simulink model "TxSteering_RxMVDR_4x4_HDL_IQ"  (R2023a)
settings: Solver=FixedStepDiscrete  StartTime=0.0  StopTime=stoptime  RelTol=1e-3
PreLoadFcn:
  | model_init
InitFcn:
  | model_init
model workspace (MAT data in the model file):
  socvcb : containers.Map (value not decoded)
values from neighbouring files (symbols this model uses):
  diagLoading = 5e-3    (= 0.005)    [model_init.m]
  dmaFIFOLength = 2^nextpow2(testSrc1.FrameLength*testSrc1.SamplesPerSymbol*2)    [model_init.m]
  fc = ConverterSampleRate*7/16    (= 860160000)    [model_init.m]
  FPGAClkRate = DataSampleRate/VectorSamplingFactor    (= 245760000)    [model_init.m]
  movavg_bitshift = nextpow2(windowSize)    [model_init.m]
  mvdrPipelineDelay = covMatDelay+movAvgDelay+matrixSolveDelay+normResponseDelay    [model_init.m]
  NCO_bits = 14    [model_init.m]
  numArrayElements = 4    [model_init.m]
  NumChan = 4    [model_init.m]
  reciprocalDelay = nextpow2(reciprocalin_dt.WordLength) + 1 + reciprocalin_dt.WordLength + 2      - strcmp(reciprocalin_dt.Signedness,'Signed') + 7    [model_init.m]
  rx_mag_delay = input_dt.WordLength + 2 + ceil(log2(NumChan)) + 1 + rx_mag_window_size    [model_init.m]
  rx_mag_inverse_delay = nextpow2(rx_mag_dt.WordLength) + 1 + rx_mag_dt.WordLength + 2 + 7    [model_init.m]
  rx_mag_sum_growth = nextpow2(rx_mag_window_size)    [model_init.m]
  rx_mag_window_size = 256    [model_init.m]
  s2mmFrameSize = testSrc1.FrameLength*testSrc1.SamplesPerSymbol*3    [model_init.m]
  testSrc1 = struct()    [model_init.m]
  testSrc2 = struct()    [model_init.m]
  windowSize = 4096    [model_init.m]
undefined symbols (not defined in the file or in its folder): Add, j, NumBits1, NumBits2, physconst, Shift
libraries: hdlsllib x29, simulink x15, embreciprocals x2, dspsrcs4 x2, dsphdlmathfun2 x1, embsystolicmatrixops x1, dsphdlsigops2 x1, commrfcorlib x1
(part 3 of 3)

== system TxSteering_RxMVDR_4x4_HDL_IQ/DUT/Rx Beamforming/MVDR HDL/Normalize Response/Set Latch ==
  S : Inport
  Logical Operator5 : Logic  Operator=OR  IconShape=distinctive  AllPortsSameDT=off  OutDataTypeStr=boolean
  Unit Delay : UnitDelay  SampleTime=-1  HasFrameUpgradeWarning=on
  Q : Outport  VectorParamsAs1DForOutWhenUnconnected=off
  wires:
  S/1 -> Logical Operator5/1
  Logical Operator5/1 -> Unit Delay/1
  Unit Delay/1 -> Logical Operator5/2, Q/1

== system TxSteering_RxMVDR_4x4_HDL_IQ/DUT/Rx Beamforming/Output Selector/PackInput/Pack Samples ==
  u : Inport
  Pack Samples Fcn : MATLAB Function  TreatAsAtomicUnit=on
  y : Outport
  wires:
  u/1 -> Pack Samples Fcn/1(u)
  Pack Samples Fcn/1(y) -> y/1

== system TxSteering_RxMVDR_4x4_HDL_IQ/DUT/Rx Beamforming/Output Selector/PackInput1/Pack Samples ==
  u : Inport
  Pack Samples Fcn : MATLAB Function  TreatAsAtomicUnit=on
  y : Outport
  wires:
  u/1 -> Pack Samples Fcn/1(u)
  Pack Samples Fcn/1(y) -> y/1

== system TxSteering_RxMVDR_4x4_HDL_IQ/DUT/Rx Beamforming/Output Selector/PackMVDR/Pack Samples ==
  u : Inport
  Pack Samples Fcn : MATLAB Function  TreatAsAtomicUnit=on
  y : Outport
  wires:
  u/1 -> Pack Samples Fcn/1(u)
  Pack Samples Fcn/1(y) -> y/1

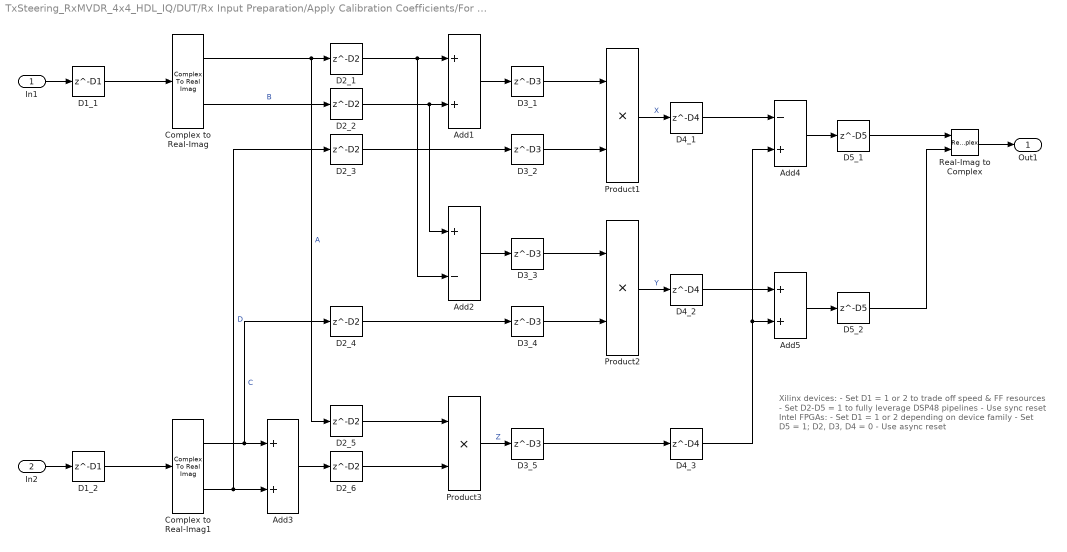
== system TxSteering_RxMVDR_4x4_HDL_IQ/DUT/Rx Input Preparation/Apply Calibration Coefficients/For Each Subsystem/HDL Complex Multiply ==
  note: Xilinx devices:
      | - Set D1 = 1 or 2 to trade off speed & FF resources
      | - Set D2-D5 = 1 to fully leverage DSP48 pipelines
      | - Use sync reset
      |
      | Intel FPGAs:
      | - Set D1 = 1 or 2 depending on device family
      | - Set D5 = 1; D2, D3, D4 = 0
      | - Use async reset
  In1 : Inport
  In2 : Inport  Port=2
  Add1 : Sum
  Add2 : Sum  Inputs=+-
  Add3 : Sum
  Add4 : Sum  Inputs=-+
  Add5 : Sum
  Complex to Real-Imag : ComplexToRealImag
  Complex to Real-Imag1 : ComplexToRealImag
  D1_1 : Delay  DelayLength=D1
  D1_2 : Delay  DelayLength=D1
  D2_{1..6} (6 alike) : Delay  DelayLength=D2
  D3_{1..5} (5 alike) : Delay  DelayLength=D3
  D4_1 : Delay  DelayLength=D4
  D4_2 : Delay  DelayLength=D4
  D4_3 : Delay  DelayLength=D4
  D5_1 : Delay  DelayLength=D5
  D5_2 : Delay  DelayLength=D5
  Product1 : Product
  Product2 : Product
  Product3 : Product
  Real-Imag to Complex : RealImagToComplex
  Out1 : Outport  VectorParamsAs1DForOutWhenUnconnected=off
  wires:
  D1_2/1 -> Complex to Real-Imag1/1
  D1_1/1 -> Complex to Real-Imag/1
  In1/1 -> D1_1/1
  D2_1/1 -> Add1/1, Add2/2
  D2_2/1 -> Add2/1, Add1/2
  D2_5/1 -> Product3/1
  D2_3/1 -> D3_2/1
  D2_4/1 -> D3_4/1
  D3_2/1 -> Product1/2
  D3_4/1 -> Product2/2
  D4_3/1 -> Add5/2, Add4/2
  D3_3/1 -> Product2/1
  D2_6/1 -> Product3/2
  D3_1/1 -> Product1/1
  Complex to Real-Imag/2 -> D2_2/1  "B"
  Complex to Real-Imag/1 -> D2_1/1, D2_5/1  "A"
  Add2/1 -> D3_3/1
  Add3/1 -> D2_6/1
  Add1/1 -> D3_1/1
  D3_5/1 -> D4_3/1
  D4_2/1 -> Add5/1
  D4_1/1 -> Add4/1
  D5_2/1 -> Real-Imag to Complex/2
  D5_1/1 -> Real-Imag to Complex/1
  Add5/1 -> D5_2/1
  Add4/1 -> D5_1/1
  Product3/1 -> D3_5/1  "Z"
  Product2/1 -> D4_2/1  "Y"
  Product1/1 -> D4_1/1  "X"
  Complex to Real-Imag1/2 -> D2_3/1, Add3/2  "D"
  Complex to Real-Imag1/1 -> D2_4/1, Add3/1  "C"
  In2/1 -> D1_2/1
  Real-Imag to Complex/1 -> Out1/1

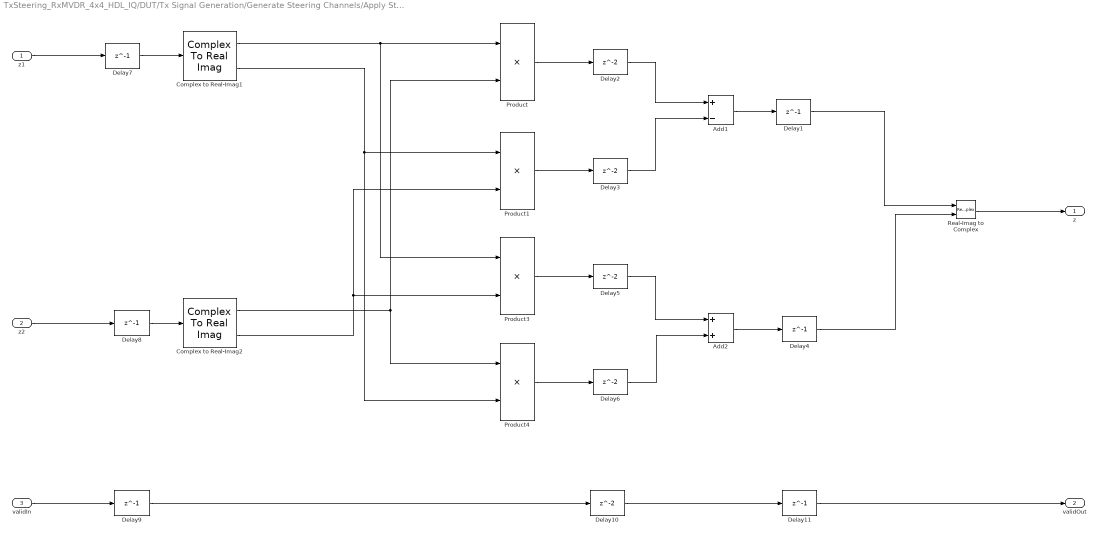
== system TxSteering_RxMVDR_4x4_HDL_IQ/DUT/Tx Signal Generation/Generate Steering Channels/Apply Steering Coefficients/HDL Complex Multiplier ==
  z1 : Inport
  z2 : Inport  Port=2
  validIn : Inport  Port=3
  Add1 : Sum  Inputs=+-
  Add2 : Sum
  Complex to Real-Imag1 : ComplexToRealImag
  Complex to Real-Imag2 : ComplexToRealImag
  Delay{1,4,7..9,11} (6 alike) : Delay  DelayLength=1  InitialCondition=0  InputProcessing=Columns as channels (frame based)
  Delay{2..3,5..6,10} (5 alike) : Delay  InitialCondition=0  InputProcessing=Columns as channels (frame based)
  Product{,1,3..4} (4 alike) : Product
  Real-Imag to Complex : RealImagToComplex
  z : Outport  VectorParamsAs1DForOutWhenUnconnected=off
  validOut : Outport  Port=2  VectorParamsAs1DForOutWhenUnconnected=off
  wires:
  Add2/1 -> Delay4/1
  Add1/1 -> Delay1/1
  Complex to Real-Imag2/2 -> Product1/2, Product3/2
  Complex to Real-Imag1/2 -> Product1/1, Product4/2
  Complex to Real-Imag2/1 -> Product/2, Product4/1
  Complex to Real-Imag1/1 -> Product/1, Product3/1
  Product/1 -> Delay2/1
  Product1/1 -> Delay3/1
  Product3/1 -> Delay5/1
  Product4/1 -> Delay6/1
  Delay2/1 -> Add1/1
  Delay3/1 -> Add1/2
  Delay6/1 -> Add2/2
  Real-Imag to Complex/1 -> z/1
  z1/1 -> Delay7/1
  z2/1 -> Delay8/1
  Delay5/1 -> Add2/1
  Delay1/1 -> Real-Imag to Complex/1
  Delay4/1 -> Real-Imag to Complex/2
  Delay7/1 -> Complex to Real-Imag1/1
  Delay8/1 -> Complex to Real-Imag2/1
  validIn/1 -> Delay9/1
  Delay9/1 -> Delay10/1
  Delay10/1 -> Delay11/1
  Delay11/1 -> validOut/1

== system TxSteering_RxMVDR_4x4_HDL_IQ/DUT/Rx Beamforming/Input Scaling/Compute Input Magnitude/Delay Enabled Synchronous/Synchronous Delay ==
  u : Inport
  E : Inport  Port=2
  Delay : Delay  DelayLength=DelayLength  InitialCondition=InitialCondition  ShowEnablePort=on
      settings: InputPortMap=u0,e6
  State Control : StateControl  StateControl=Synchronous
  y : Outport
  wires:
  Delay/1 -> y/1
  E/1 -> Delay/2
  u/1 -> Delay/1

== system TxSteering_RxMVDR_4x4_HDL_IQ/DUT/Rx Beamforming/MVDR HDL/Compute Weight Vector/Serialize Input Data/Output Selector ==
  idx : Inport
  first : Inport  Port=2
  dataIn : Inport  Port=3
  Multiport Switch : MultiPortSwitch  DataPortOrder=Zero-based contiguous  Inputs=4  zeroidx=on  SaturateOnIntegerOverflow=off  InputSameDT=off
  Row 1 : Selector  NumberOfDimensions=2  InputPortWidth=3  IndexOptions=Index vector (dialog),Select all  Indices=1,1  OutputSizes=1,1
  Row 2 : Selector  NumberOfDimensions=2  InputPortWidth=3  IndexOptions=Index vector (dialog),Select all  Indices=2,1  OutputSizes=1,1
  Row 3 : Selector  NumberOfDimensions=2  InputPortWidth=3  IndexOptions=Index vector (dialog),Select all  Indices=3,1  OutputSizes=1,1
  Row 4 : Selector  NumberOfDimensions=2  InputPortWidth=3  IndexOptions=Index vector (dialog),Select all  Indices=4,1  OutputSizes=1,1
  Unit Delay Enabled Synchronous : hdlsllib/Discrete/Unit Delay Enabled Synchronous  InitialCondition=0.0  SampleTime=-1
  dataOut : Outport
  wires:
  Row 1/1 -> Multiport Switch/2
  Row 4/1 -> Multiport Switch/5
  Unit Delay Enabled Synchronous/1 -> Row 4/1, Row 3/1, Row 2/1
  dataIn/1 -> Unit Delay Enabled Synchronous/1, Row 1/1
  Row 2/1 -> Multiport Switch/3
  idx/1 -> Multiport Switch/1
  Row 3/1 -> Multiport Switch/4
  Multiport Switch/1 -> dataOut/1
  first/1 -> Unit Delay Enabled Synchronous/2

== system TxSteering_RxMVDR_4x4_HDL_IQ/DUT/Rx Beamforming/MVDR HDL/Compute Weight Vector/Serialize Input Data/Output Selector1 ==
  idx : Inport
  first : Inport  Port=2
  dataIn : Inport  Port=3
  Multiport Switch : MultiPortSwitch  DataPortOrder=Zero-based contiguous  Inputs=4  zeroidx=on  SaturateOnIntegerOverflow=off  InputSameDT=off
  Row 1 : Selector  NumberOfDimensions=2  InputPortWidth=3  IndexOptions=Index vector (dialog),Select all  Indices=1,1  OutputSizes=1,1
  Row 2 : Selector  NumberOfDimensions=2  InputPortWidth=3  IndexOptions=Index vector (dialog),Select all  Indices=2,1  OutputSizes=1,1
  Row 3 : Selector  NumberOfDimensions=2  InputPortWidth=3  IndexOptions=Index vector (dialog),Select all  Indices=3,1  OutputSizes=1,1
  Row 4 : Selector  NumberOfDimensions=2  InputPortWidth=3  IndexOptions=Index vector (dialog),Select all  Indices=4,1  OutputSizes=1,1
  Unit Delay Enabled Synchronous : hdlsllib/Discrete/Unit Delay Enabled Synchronous  InitialCondition=0.0  SampleTime=-1
  dataOut : Outport
  wires:
  first/1 -> Unit Delay Enabled Synchronous/2
  Multiport Switch/1 -> dataOut/1
  Row 3/1 -> Multiport Switch/4
  idx/1 -> Multiport Switch/1
  Row 2/1 -> Multiport Switch/3
  dataIn/1 -> Row 1/1, Unit Delay Enabled Synchronous/1
  Unit Delay Enabled Synchronous/1 -> Row 2/1, Row 3/1, Row 4/1
  Row 4/1 -> Multiport Switch/5
  Row 1/1 -> Multiport Switch/2

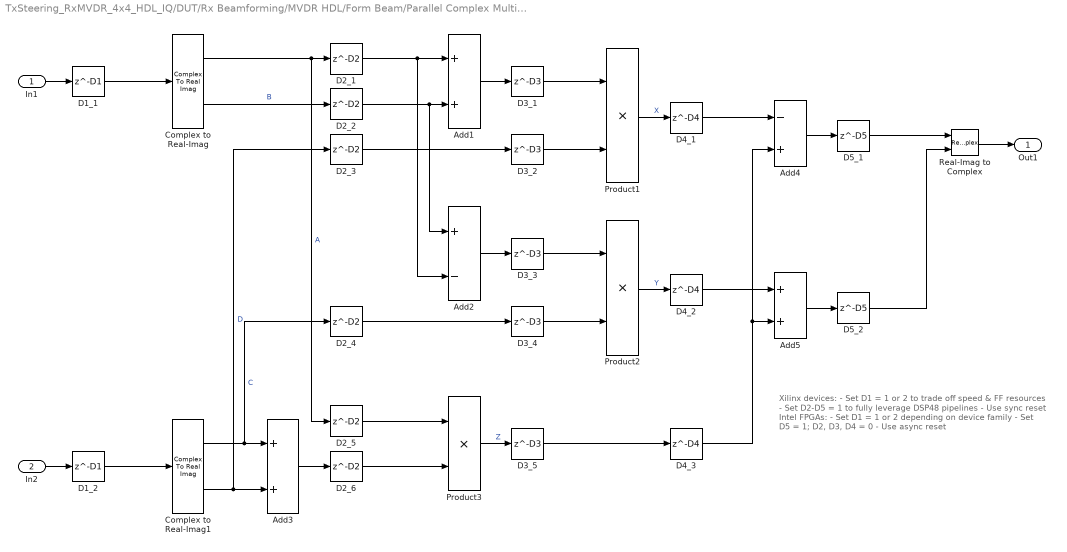
== system TxSteering_RxMVDR_4x4_HDL_IQ/DUT/Rx Beamforming/MVDR HDL/Form Beam/Parallel Complex Multiply/HDL Complex Multiply ==
  note: Xilinx devices:
      | - Set D1 = 1 or 2 to trade off speed & FF resources
      | - Set D2-D5 = 1 to fully leverage DSP48 pipelines
      | - Use sync reset
      |
      | Intel FPGAs:
      | - Set D1 = 1 or 2 depending on device family
      | - Set D5 = 1; D2, D3, D4 = 0
      | - Use async reset
  In1 : Inport
  In2 : Inport  Port=2
  Add1 : Sum
  Add2 : Sum  Inputs=+-
  Add3 : Sum
  Add4 : Sum  Inputs=-+
  Add5 : Sum
  Complex to Real-Imag : ComplexToRealImag
  Complex to Real-Imag1 : ComplexToRealImag
  D1_1 : Delay  DelayLength=D1
  D1_2 : Delay  DelayLength=D1
  D2_{1..6} (6 alike) : Delay  DelayLength=D2
  D3_{1..5} (5 alike) : Delay  DelayLength=D3
  D4_1 : Delay  DelayLength=D4
  D4_2 : Delay  DelayLength=D4
  D4_3 : Delay  DelayLength=D4
  D5_1 : Delay  DelayLength=D5
  D5_2 : Delay  DelayLength=D5
  Product1 : Product
  Product2 : Product
  Product3 : Product
  Real-Imag to Complex : RealImagToComplex
  Out1 : Outport  VectorParamsAs1DForOutWhenUnconnected=off
  wires:
  Real-Imag to Complex/1 -> Out1/1
  In2/1 -> D1_2/1
  Complex to Real-Imag1/1 -> Add3/1, D2_4/1  "C"
  Complex to Real-Imag1/2 -> Add3/2, D2_3/1  "D"
  Product1/1 -> D4_1/1  "X"
  Product2/1 -> D4_2/1  "Y"
  Product3/1 -> D3_5/1  "Z"
  Add4/1 -> D5_1/1
  Add5/1 -> D5_2/1
  D5_1/1 -> Real-Imag to Complex/1
  D5_2/1 -> Real-Imag to Complex/2
  D4_1/1 -> Add4/1
  D4_2/1 -> Add5/1
  D3_5/1 -> D4_3/1
  Add1/1 -> D3_1/1
  Add3/1 -> D2_6/1
  Add2/1 -> D3_3/1
  Complex to Real-Imag/1 -> D2_5/1, D2_1/1  "A"
  Complex to Real-Imag/2 -> D2_2/1  "B"
  D3_1/1 -> Product1/1
  D2_6/1 -> Product3/2
  D3_3/1 -> Product2/1
  D4_3/1 -> Add4/2, Add5/2
  D3_4/1 -> Product2/2
  D3_2/1 -> Product1/2
  D2_4/1 -> D3_4/1
  D2_3/1 -> D3_2/1
  D2_5/1 -> Product3/1
  D2_2/1 -> Add1/2, Add2/1
  D2_1/1 -> Add2/2, Add1/1
  In1/1 -> D1_1/1
  D1_1/1 -> Complex to Real-Imag/1
  D1_2/1 -> Complex to Real-Imag1/1

== system TxSteering_RxMVDR_4x4_HDL_IQ/DUT/Rx Beamforming/MVDR HDL/Form Covariance Matrix/Matrix Multiply Partitioned/Partition x_conj ==
  x : Inport
  x_conj : Inport  Port=2  Partition=on  PartitionDimension=1  PartitionWidth=1  PartitionOffset=0
  For Each : ForEach  DisableCoverage=on
  Partition x : Subsystem  TreatAsAtomicUnit=on
  C : Outport  ConcatenationDimension=1
  wires:
  x_conj/1 -> Partition x/2(x_conj_elem)
  x/1 -> Partition x/1(x)
  Partition x/1(C_col) -> C/1

== system TxSteering_RxMVDR_4x4_HDL_IQ/DUT/Rx Beamforming/MVDR HDL/Moving Average/Window Delay/Delay Enabled Synchronous RAM Based ==
  u : Inport
  E : Inport  Port=2
  Add : Sum  Inputs=++-  OutDataTypeStr=Inherit: Same as accumulator
  Constant1 : Constant  OutDataTypeStr=Inherit: Inherit via back propagation  SampleTime=-1
  Constant2 : Constant  Value=delay  OutDataTypeStr=Inherit: Inherit via back propagation  SampleTime=-1
  HDL Counter : hdlsllib/Sources/HDL Counter  CountType=Free running  CountInit=0  CountStep=1  CountMax=25  CountFromType=Initial value  CountFrom=0  CountResetPort=off  CountLoadPort=off  CountEnbPort=on  CountDirPort=off  CountHitOutputPort=off  CountDataType=Unsigned  CountWordLen=addrWidth  CountFracLen=0  CountSampTime=-1
  Simple Dual Port RAM System : hdlsllib/HDL RAMs/Simple Dual Port RAM System  RAMType=Simple dual port  WriteOutputValue=New data  RAMInitialValue=0  SimulateUsing=Code generation
  Switch1 : Switch  Criteria=u2 ~= 0  SaturateOnIntegerOverflow=off  InputSameDT=off
  Zero on Initial Delay : Subsystem
  out_prev : hdlsllib/Discrete/Unit Delay Enabled Synchronous  InitialCondition=0.0  SampleTime=-1
  read_prev : Delay  DelayLength=1
  y : Outport
  wires:
  read_prev/1 -> Switch1/2, out_prev/2
  Zero on Initial Delay/1(dout) -> Switch1/1, out_prev/1
  Simple Dual Port RAM System/1 -> Zero on Initial Delay/1(ram_dout)
  E/1 -> HDL Counter/1, Zero on Initial Delay/2(en), read_prev/1, Simple Dual Port RAM System/3
  out_prev/1 -> Switch1/3
  Switch1/1 -> y/1
  Constant2/1 -> Add/3
  Constant1/1 -> Add/2
  u/1 -> Simple Dual Port RAM System/1
  Add/1 -> Simple Dual Port RAM System/4
  HDL Counter/1 -> Add/1, Simple Dual Port RAM System/2

== system TxSteering_RxMVDR_4x4_HDL_IQ/DUT/Rx Beamforming/MVDR HDL/Normalize Response/MVDR Weight Update/Inner Product ==
  sv : Inport
  wp : Inport  Port=2
  validIn : Inport  Port=3
  Complex to Real-Imag : ComplexToRealImag  Output=Real
  Conjugate : Math  Operator=conj  SignedPower=on  RndMeth=Zero
  Data Type Conversion : DataTypeConversion  OutDataTypeStr=reciprocalin_dt  SaturateOnIntegerOverflow=off  RndMeth=Floor
  Delay : Delay  DelayLength=1
  Delay1 : Delay  DelayLength=6
  Delay2 : Delay  DelayLength=ceil(log2(numArrayElements))
  Delay4 : Delay  DelayLength=1
  Element-wise complex product : Subsystem  TreatAsAtomicUnit=on
  To Workspace : ToWorkspace  VariableName=norm_mag  SampleTime=-1
      settings: Save2DSignal=2-D array (concatenate along first dimension)
  To Workspace1 : ToWorkspace  VariableName=norm_mag_valid  SampleTime=-1
      settings: Save2DSignal=2-D array (concatenate along first dimension)
  Tree Sum with Distributed Pipelining : Subsystem
  y : Outport
  validOut : Outport  Port=2
  wires:
  sv/1 -> Conjugate/1
  validIn/1 -> Delay1/1
  Delay1/1 -> Delay4/1
  Delay4/1 -> Delay2/1
  wp/1 -> Element-wise complex product/1(u)
  Delay/1 -> Tree Sum with Distributed Pipelining/1(In1)
  Complex to Real-Imag/1 -> Data Type Conversion/1
  Element-wise complex product/1(y) -> Delay/1
  Delay2/1 -> validOut/1, To Workspace1/1
  Tree Sum with Distributed Pipelining/1(Out1) -> Complex to Real-Imag/1
  Data Type Conversion/1 -> y/1, To Workspace/1
  Conjugate/1 -> Element-wise complex product/2(v)

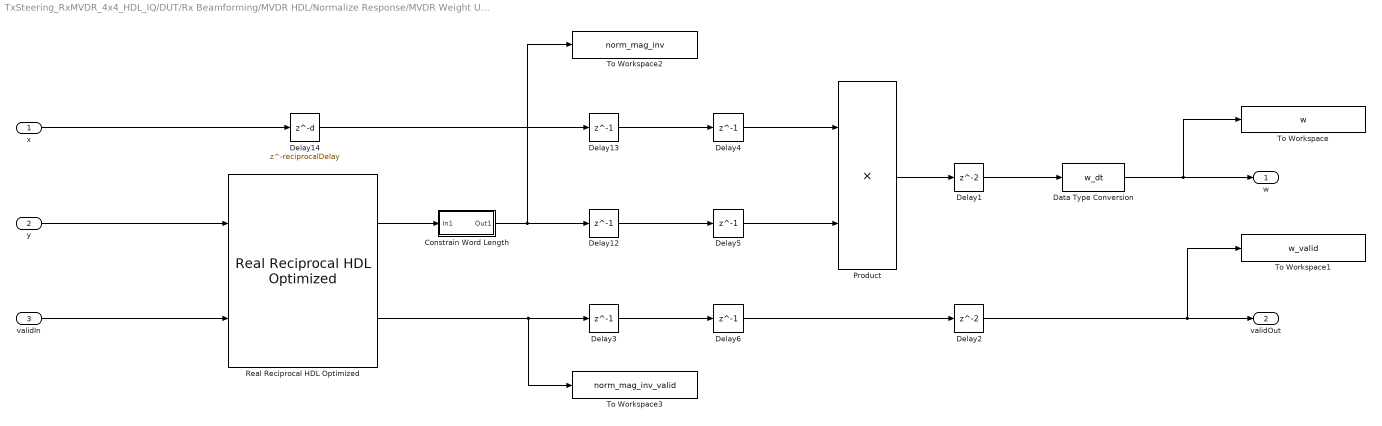
== system TxSteering_RxMVDR_4x4_HDL_IQ/DUT/Rx Beamforming/MVDR HDL/Normalize Response/MVDR Weight Update/Vector // Scalar Divide ==
  x : Inport
  y : Inport  Port=2
  validIn : Inport  Port=3
  Constrain Word Length : Subsystem  mask(Constrain Word Length){WL=18}
      mask prompts: WL "Maximum word length:"
      mask help: Output word length will not exceed the specified value.
      mask Display: fprintf('WL <= %d',WL);
  Data Type Conversion : DataTypeConversion  OutDataTypeStr=w_dt  SaturateOnIntegerOverflow=off  RndMeth=Floor
  Delay1 : Delay
  Delay{3..6,12..13} (6 alike) : Delay  DelayLength=1
  Delay14 : Delay  DelayLength=reciprocalDelay
  Delay2 : Delay
  Product : Product
  Real Reciprocal HDL Optimized : embreciprocals/Real Reciprocal HDL Optimized  OutputType=reciprocalout_dt
      settings: LibrarySourceBlock=embeddedMatrixLib/Math Operations/Real Reciprocal HDL Optimized
  To Workspace : ToWorkspace  VariableName=w  SampleTime=-1
      settings: Save2DSignal=2-D array (concatenate along first dimension)
  To Workspace1 : ToWorkspace  VariableName=w_valid  SampleTime=-1
      settings: Save2DSignal=2-D array (concatenate along first dimension)
  To Workspace2 : ToWorkspace  VariableName=norm_mag_inv  SampleTime=-1
      settings: Save2DSignal=2-D array (concatenate along first dimension)
  To Workspace3 : ToWorkspace  VariableName=norm_mag_inv_valid  SampleTime=-1
      settings: Save2DSignal=2-D array (concatenate along first dimension)
  w : Outport
  validOut : Outport  Port=2
  wires:
  y/1 -> Real Reciprocal HDL Optimized/1
  Real Reciprocal HDL Optimized/1 -> Constrain Word Length/1(In1)
  validIn/1 -> Real Reciprocal HDL Optimized/2
  Product/1 -> Delay1/1
  x/1 -> Delay14/1
  Delay14/1 -> Delay13/1
  Constrain Word Length/1(Out1) -> To Workspace2/1, Delay12/1
  Real Reciprocal HDL Optimized/2 -> To Workspace3/1, Delay3/1
  Delay2/1 -> To Workspace1/1, validOut/1
  Delay1/1 -> Data Type Conversion/1
  Data Type Conversion/1 -> To Workspace/1, w/1
  Delay4/1 -> Product/1
  Delay13/1 -> Delay4/1
  Delay5/1 -> Product/2
  Delay12/1 -> Delay5/1
  Delay3/1 -> Delay6/1
  Delay6/1 -> Delay2/1

== system TxSteering_RxMVDR_4x4_HDL_IQ/DUT/Rx Beamforming/MVDR HDL/Form Covariance Matrix/Matrix Multiply Partitioned/Partition x_conj/Partition x ==
  x : Inport  Partition=on  PartitionDimension=1  PartitionWidth=1  PartitionOffset=0
  x_conj_elem : Inport  Port=2
  For Each : ForEach  DisableCoverage=on
  HDL Complex Multiply : Subsystem  mask(HDL Complex Multiplier (3 Multiply, 5 Add)){D1=2, D2=1, D3=1, D4=1, D5=1}
      mask help:
      | Xilinx devices:
      | - Set D1 = 1 or 2 to trade off speed & FF resources
      | - Set D2-D5 = 1 to fully leverage DSP48 pipelines
      | - Use sync reset
      |
      | Intel FPGAs:
      | - Set D1 = 1 or 2 depending on device family
      | - Set D5 = 1; D2, D3, D4 = 0
      | - Use async reset
      mask init:
      | delay = D1+D2+D3+D4+D5;
      mask Display:
      | fprintf('Delay=%d',delay);
      | port_label('input',1,'z1');
      | port_label('input',2,'z2');
  C_col : Outport  ConcatenationDimension=1
  wires:
  x/1 -> HDL Complex Multiply/1(In1)
  x_conj_elem/1 -> HDL Complex Multiply/2(In2)
  HDL Complex Multiply/1(Out1) -> C_col/1

== system TxSteering_RxMVDR_4x4_HDL_IQ/DUT/Rx Beamforming/MVDR HDL/Moving Average/Window Delay/Delay Enabled Synchronous RAM Based/Zero on Initial Delay ==
  ram_dout : Inport
  en : Inport  Port=2
  AND : Logic  IconShape=distinctive  AllPortsSameDT=off  OutDataTypeStr=boolean
  Compare To Constant : simulink/Logic and Bit Operations/Compare To Constant  relop===  const=delay  OutDataTypeStr=boolean
  HDL Counter1 : hdlsllib/Sources/HDL Counter  CountType=Free running  CountInit=0  CountStep=1  CountMax=25  CountFromType=Initial value  CountFrom=0  CountResetPort=off  CountLoadPort=off  CountEnbPort=on  CountDirPort=off  CountHitOutputPort=off  CountDataType=Unsigned  CountWordLen=addrWidth  CountFracLen=0  CountSampTime=-1
  NOT : Logic  Operator=NOT  IconShape=distinctive  AllPortsSameDT=off  OutDataTypeStr=boolean
  Switch : Switch  Criteria=u2 ~= 0  SaturateOnIntegerOverflow=off  InputSameDT=off
  Zeros Like : MATLAB Function  TreatAsAtomicUnit=on  mask(Zeros Like){matchInputSize=on, outputSizeUser=[1 1]}
      mask prompts: matchInputSize "Match input size?"; outputSizeUser "Output size:"
      mask help: Creates a constant 0 signal with the same datatype as the input. Optionally match the size of the input or specify the output size.
      mask init:
      | if isscalar(outputSizeUser)
      |     outputSize = [outputSizeUser 1];
      | else
      |     outputSize = outputSizeUser;
      | end
  dout : Outport
  wires:
  en/1 -> AND/1
  ram_dout/1 -> Switch/1, Zeros Like/1(u)
  AND/1 -> HDL Counter1/1
  Zeros Like/1(y) -> Switch/3
  NOT/1 -> AND/2
  Compare To Constant/1 -> NOT/1, Switch/2
  HDL Counter1/1 -> Compare To Constant/1
  Switch/1 -> dout/1

== system TxSteering_RxMVDR_4x4_HDL_IQ/DUT/Rx Beamforming/MVDR HDL/Normalize Response/MVDR Weight Update/Inner Product/Element-wise complex product ==
  u : Inport  Partition=on  PartitionDimension=1  PartitionWidth=1  PartitionOffset=0
  v : Inport  Port=2  Partition=on  PartitionDimension=1  PartitionWidth=1  PartitionOffset=0
  For Each : ForEach  DisableCoverage=on
  HDL Complex Multiply : Subsystem  mask(HDL Complex Multiplier (3 Multiply, 5 Add)){D1=2, D2=1, D3=1, D4=1, D5=1}
      mask help:
      | Xilinx devices:
      | - Set D1 = 1 or 2 to trade off speed & FF resources
      | - Set D2-D5 = 1 to fully leverage DSP48 pipelines
      | - Use sync reset
      |
      | Intel FPGAs:
      | - Set D1 = 1 or 2 depending on device family
      | - Set D5 = 1; D2, D3, D4 = 0
      | - Use async reset
      mask init:
      | delay = D1+D2+D3+D4+D5;
      mask Display:
      | fprintf('Pipelined\nComplex Multiply\nLatency=%d',delay);
      | port_label('input',1,'z1');
      | port_label('input',2,'z2');
  y : Outport  ConcatenationDimension=1
  wires:
  v/1 -> HDL Complex Multiply/2(In2)
  u/1 -> HDL Complex Multiply/1(In1)
  HDL Complex Multiply/1(Out1) -> y/1

== system TxSteering_RxMVDR_4x4_HDL_IQ/DUT/Rx Beamforming/MVDR HDL/Normalize Response/MVDR Weight Update/Inner Product/Tree Sum with Distributed Pipelining ==
  In1 : Inport
  Delay3 : Delay  DelayLength=ceil(log2(numArrayElements))
  Tree Sum of Elements : Sum  Inputs=+  OutDataTypeStr=Inherit: Same as first input  LockScale=on
  Out1 : Outport
  wires:
  Delay3/1 -> Out1/1
  In1/1 -> Tree Sum of Elements/1
  Tree Sum of Elements/1 -> Delay3/1

== system TxSteering_RxMVDR_4x4_HDL_IQ/DUT/Rx Beamforming/MVDR HDL/Normalize Response/MVDR Weight Update/Vector // Scalar Divide/Constrain Word Length ==
  In1 : Inport
  Constant : Constant  Value=0  OutDataTypeStr=fixdt(0,WL,0)  SampleTime=-1
  Data Type Propagation : simulink/Signal Attributes/Data Type Propagation  PropDataType=fixdt(1, 16)  IfRefDouble=double  IfRefSingle=single  IsSigned=IsSigned1  NumBitsBase=min([NumBits1 NumBits2])  NumBitsMult=1  NumBitsAdd=0  NumBitsAllowFinal=1:128  PropScaling=2^-10  ValuesUsedBestPrec=[5 -7]  SlopeBase=PosRange1  SlopeMult=1  SlopeAdd=0  BiasBase=Bias1  BiasMult=1  BiasAdd=0
  Data Type Conversion : DataTypeConversion  SaturateOnIntegerOverflow=off  RndMeth=Floor
  Out1 : Outport
  wires:
  Constant/1 -> Data Type Propagation/2
  Data Type Conversion/1 -> Out1/1, Data Type Propagation/3
  In1/1 -> Data Type Conversion/1, Data Type Propagation/1

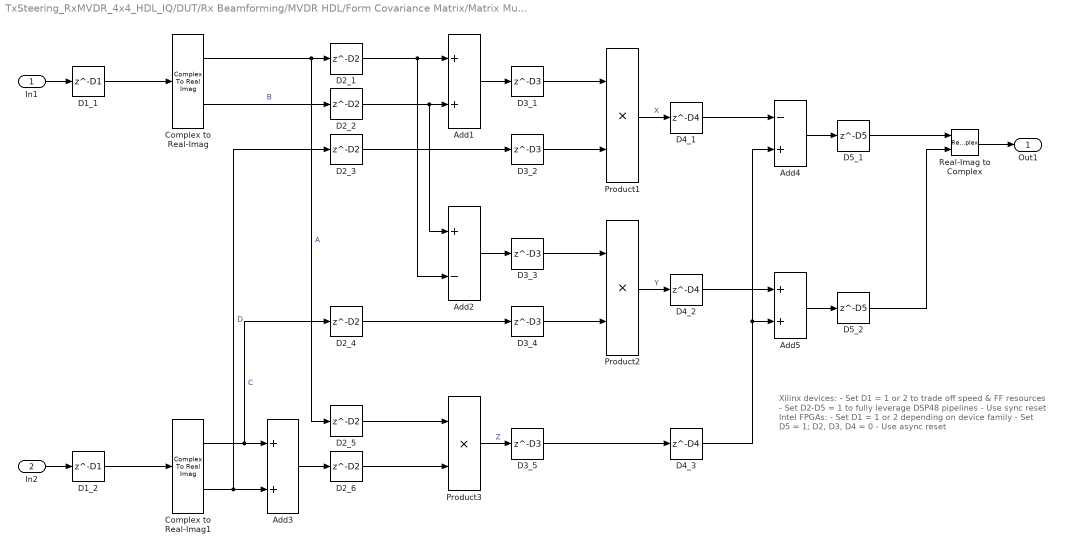
== system TxSteering_RxMVDR_4x4_HDL_IQ/DUT/Rx Beamforming/MVDR HDL/Form Covariance Matrix/Matrix Multiply Partitioned/Partition x_conj/Partition x/HDL Complex Multiply ==
  note: Xilinx devices:
      | - Set D1 = 1 or 2 to trade off speed & FF resources
      | - Set D2-D5 = 1 to fully leverage DSP48 pipelines
      | - Use sync reset
      |
      | Intel FPGAs:
      | - Set D1 = 1 or 2 depending on device family
      | - Set D5 = 1; D2, D3, D4 = 0
      | - Use async reset
  In1 : Inport
  In2 : Inport  Port=2
  Add1 : Sum
  Add2 : Sum  Inputs=+-
  Add3 : Sum
  Add4 : Sum  Inputs=-+
  Add5 : Sum
  Complex to Real-Imag : ComplexToRealImag
  Complex to Real-Imag1 : ComplexToRealImag
  D1_1 : Delay  DelayLength=D1
  D1_2 : Delay  DelayLength=D1
  D2_{1..6} (6 alike) : Delay  DelayLength=D2
  D3_{1..5} (5 alike) : Delay  DelayLength=D3
  D4_1 : Delay  DelayLength=D4
  D4_2 : Delay  DelayLength=D4
  D4_3 : Delay  DelayLength=D4
  D5_1 : Delay  DelayLength=D5
  D5_2 : Delay  DelayLength=D5
  Product1 : Product
  Product2 : Product
  Product3 : Product
  Real-Imag to Complex : RealImagToComplex
  Out1 : Outport  VectorParamsAs1DForOutWhenUnconnected=off
  wires:
  Real-Imag to Complex/1 -> Out1/1
  In2/1 -> D1_2/1
  Complex to Real-Imag1/1 -> Add3/1, D2_4/1  "C"
  Complex to Real-Imag1/2 -> Add3/2, D2_3/1  "D"
  Product1/1 -> D4_1/1  "X"
  Product2/1 -> D4_2/1  "Y"
  Product3/1 -> D3_5/1  "Z"
  Add4/1 -> D5_1/1
  Add5/1 -> D5_2/1
  D5_1/1 -> Real-Imag to Complex/1
  D5_2/1 -> Real-Imag to Complex/2
  D4_1/1 -> Add4/1
  D4_2/1 -> Add5/1
  D3_5/1 -> D4_3/1
  Add1/1 -> D3_1/1
  Add3/1 -> D2_6/1
  Add2/1 -> D3_3/1
  Complex to Real-Imag/1 -> D2_5/1, D2_1/1  "A"
  Complex to Real-Imag/2 -> D2_2/1  "B"
  D3_1/1 -> Product1/1
  D2_6/1 -> Product3/2
  D3_3/1 -> Product2/1
  D4_3/1 -> Add4/2, Add5/2
  D3_4/1 -> Product2/2
  D3_2/1 -> Product1/2
  D2_4/1 -> D3_4/1
  D2_3/1 -> D3_2/1
  D2_5/1 -> Product3/1
  D2_2/1 -> Add1/2, Add2/1
  D2_1/1 -> Add2/2, Add1/1
  In1/1 -> D1_1/1
  D1_1/1 -> Complex to Real-Imag/1
  D1_2/1 -> Complex to Real-Imag1/1

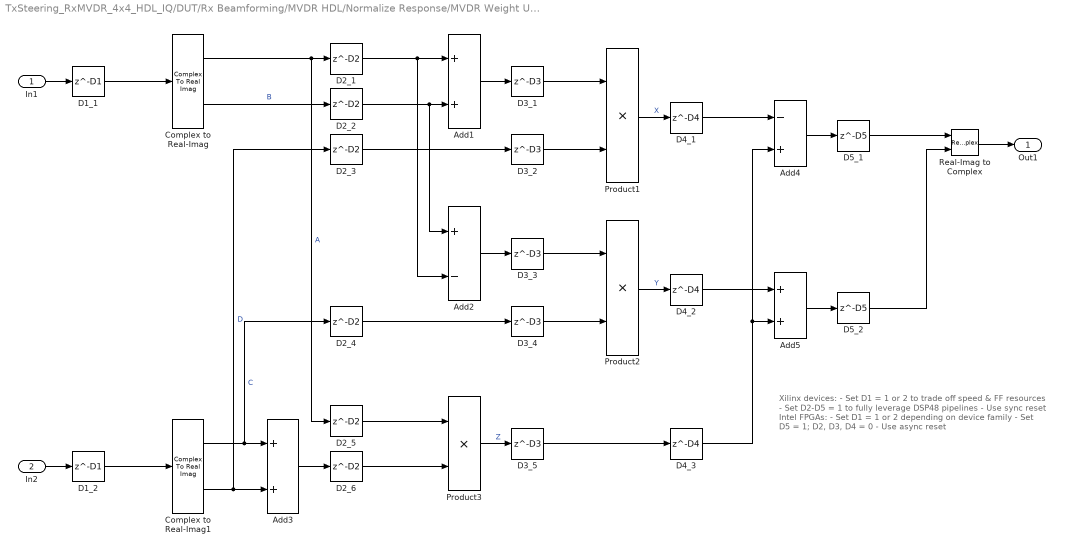
== system TxSteering_RxMVDR_4x4_HDL_IQ/DUT/Rx Beamforming/MVDR HDL/Normalize Response/MVDR Weight Update/Inner Product/Element-wise complex product/HDL Complex Multiply ==
  note: Xilinx devices:
      | - Set D1 = 1 or 2 to trade off speed & FF resources
      | - Set D2-D5 = 1 to fully leverage DSP48 pipelines
      | - Use sync reset
      |
      | Intel FPGAs:
      | - Set D1 = 1 or 2 depending on device family
      | - Set D5 = 1; D2, D3, D4 = 0
      | - Use async reset
  In1 : Inport
  In2 : Inport  Port=2
  Add1 : Sum
  Add2 : Sum  Inputs=+-
  Add3 : Sum
  Add4 : Sum  Inputs=-+
  Add5 : Sum
  Complex to Real-Imag : ComplexToRealImag
  Complex to Real-Imag1 : ComplexToRealImag
  D1_1 : Delay  DelayLength=D1
  D1_2 : Delay  DelayLength=D1
  D2_{1..6} (6 alike) : Delay  DelayLength=D2
  D3_{1..5} (5 alike) : Delay  DelayLength=D3
  D4_1 : Delay  DelayLength=D4
  D4_2 : Delay  DelayLength=D4
  D4_3 : Delay  DelayLength=D4
  D5_1 : Delay  DelayLength=D5
  D5_2 : Delay  DelayLength=D5
  Product1 : Product
  Product2 : Product
  Product3 : Product
  Real-Imag to Complex : RealImagToComplex
  Out1 : Outport  VectorParamsAs1DForOutWhenUnconnected=off
  wires:
  D1_2/1 -> Complex to Real-Imag1/1
  D1_1/1 -> Complex to Real-Imag/1
  In1/1 -> D1_1/1
  D2_1/1 -> Add1/1, Add2/2
  D2_2/1 -> Add2/1, Add1/2
  D2_5/1 -> Product3/1
  D2_3/1 -> D3_2/1
  D2_4/1 -> D3_4/1
  D3_2/1 -> Product1/2
  D3_4/1 -> Product2/2
  D4_3/1 -> Add5/2, Add4/2
  D3_3/1 -> Product2/1
  D2_6/1 -> Product3/2
  D3_1/1 -> Product1/1
  Complex to Real-Imag/2 -> D2_2/1  "B"
  Complex to Real-Imag/1 -> D2_1/1, D2_5/1  "A"
  Add2/1 -> D3_3/1
  Add3/1 -> D2_6/1
  Add1/1 -> D3_1/1
  D3_5/1 -> D4_3/1
  D4_2/1 -> Add5/1
  D4_1/1 -> Add4/1
  D5_2/1 -> Real-Imag to Complex/2
  D5_1/1 -> Real-Imag to Complex/1
  Add5/1 -> D5_2/1
  Add4/1 -> D5_1/1
  Product3/1 -> D3_5/1  "Z"
  Product2/1 -> D4_2/1  "Y"
  Product1/1 -> D4_1/1  "X"
  Complex to Real-Imag1/2 -> D2_3/1, Add3/2  "D"
  Complex to Real-Imag1/1 -> D2_4/1, Add3/1  "C"
  In2/1 -> D1_2/1
  Real-Imag to Complex/1 -> Out1/1

== matlab function TxSteering_RxMVDR_4x4_HDL_IQ/DUT/Rx Beamforming/Output Selector/PackInput1/Pack Samples/Pack Samples Fcn ==
  settings: fimath=hdlfimath;
  data: u input; y output; is_complex parameter
function y = pack_samples(u,is_complex)
%#codegen

if is_complex
    y = pack_complex(u);
else
    y = pack_real(u);
end

end

function y = pack_real(u)

    assert(isreal(u),'Expected input to be real');
    
    N = coder.const(numel(u));
    
    temp = coder.nullcopy((cast_to_fi(zeros([N 1],'like',u))));
    
    coder.unroll();
    for ii=N:-1:1
        temp(N-ii+1) = u(ii);
    end
    
    y = bitconcat(temp);

end

function y = pack_complex(u)

    assert(~isreal(u),'Expected input to be complex');
    
    N = coder.const(numel(u));
    
    temp = coder.nullcopy((cast_to_fi(zeros([N*2 1],'like',real(u)))));
    
    % Interleave real/imag
    coder.unroll();
    for ii=N:-1:1
        temp((ii-1)*2+2) = real(u(N-ii+1));
        temp((ii-1)*2+1) = imag(u(N-ii+1));
    end
    
    y = bitconcat(temp);

end

== matlab function TxSteering_RxMVDR_4x4_HDL_IQ/DUT/Rx Beamforming/MVDR HDL/Diagonal Loading/Generate Loading Eye Matrix ==
  data: in input; out output; numArrayElements parameter
function out = gen_eye(in,numArrayElements)

temp = zeros([numArrayElements numArrayElements],'like',in);
coder.unroll();
for ii=1:numArrayElements
    temp(ii,ii) = in;
end

out = temp;

== matlab function TxSteering_RxMVDR_4x4_HDL_IQ/DUT/Combine Steering Coeff Regs/Deinterleave Complex/deinterleave_complex_fcn ==
  settings: fimath=hdlfimath
  data: u input; y output
function y = deinterleave_complex(u)
%#codegen

N = coder.const(numel(u));

assert(isreal(u), 'Expected input to be real.');

temp = coder.nullcopy((cast_to_fi(complex(zeros([N/2 1],'like',u)))));

coder.unroll();
for ii=1:N/2
    temp(ii) = complex(u((ii-1)*2+1),u((ii-1)*2+2));
end

y = temp;

== matlab function TxSteering_RxMVDR_4x4_HDL_IQ/DUT/Combine Steering Coeff Regs/Deinterleave Complex1/deinterleave_complex_fcn ==
  settings: fimath=hdlfimath
  data: u input; y output
function y = deinterleave_complex(u)
%#codegen

N = coder.const(numel(u));

assert(isreal(u), 'Expected input to be real.');

temp = coder.nullcopy((cast_to_fi(complex(zeros([N/2 1],'like',u)))));

coder.unroll();
for ii=1:N/2
    temp(ii) = complex(u((ii-1)*2+1),u((ii-1)*2+2));
end

y = temp;

== matlab function TxSteering_RxMVDR_4x4_HDL_IQ/DUT/Rx Beamforming/Interleave Complex /interleave_complex_fcn ==
  settings: fimath=hdlfimath
  data: u input; y output
function y = interleave_complex(u)
%#codegen

assert(~isreal(u),'Expected input to be complex');

N = coder.const(numel(u));

temp = coder.nullcopy((cast_to_fi(zeros([N*2 1],'like',real(u)))));

coder.unroll();
for ii=1:N
    temp((ii-1)*2+1) = real(u(ii));
    temp((ii-1)*2+2) = imag(u(ii));
end

y = temp;

== matlab function TxSteering_RxMVDR_4x4_HDL_IQ/DUT/Rx Beamforming/Deinterleave Complex/deinterleave_complex_fcn ==
  settings: fimath=hdlfimath
  data: u input; y output
function y = deinterleave_complex(u)
%#codegen

N = coder.const(numel(u));

assert(isreal(u), 'Expected input to be real.');

temp = coder.nullcopy((cast_to_fi(complex(zeros([N/2 1],'like',u)))));

coder.unroll();
for ii=1:N/2
    temp(ii) = complex(u((ii-1)*2+1),u((ii-1)*2+2));
end

y = temp;

== matlab function TxSteering_RxMVDR_4x4_HDL_IQ/Software Interface Behavioral/GenSteeringCoeffs Tx Source 1/Interleave Complex 3/interleave_complex_fcn ==
  settings: fimath=hdlfimath
  data: u input; y output
function y = interleave_complex(u)
%#codegen

assert(~isreal(u),'Expected input to be complex');

N = coder.const(numel(u));

temp = coder.nullcopy((cast_to_fi(zeros([N*2 1],'like',real(u)))));

coder.unroll();
for ii=1:N
    temp((ii-1)*2+1) = real(u(ii));
    temp((ii-1)*2+2) = imag(u(ii));
end

y = temp;

== matlab function TxSteering_RxMVDR_4x4_HDL_IQ/Software Interface Behavioral/GenSteeringCoeffs Tx Source 2/Interleave Complex 3/interleave_complex_fcn ==
  settings: fimath=hdlfimath
  data: u input; y output
function y = interleave_complex(u)
%#codegen

assert(~isreal(u),'Expected input to be complex');

N = coder.const(numel(u));

temp = coder.nullcopy((cast_to_fi(zeros([N*2 1],'like',real(u)))));

coder.unroll();
for ii=1:N
    temp((ii-1)*2+1) = real(u(ii));
    temp((ii-1)*2+2) = imag(u(ii));
end

y = temp;

== matlab function TxSteering_RxMVDR_4x4_HDL_IQ/Software Interface Behavioral/GenSteeringCoeffs Rx/Interleave Complex 3/interleave_complex_fcn ==
  settings: fimath=hdlfimath
  data: u input; y output
function y = interleave_complex(u)
%#codegen

assert(~isreal(u),'Expected input to be complex');

N = coder.const(numel(u));

temp = coder.nullcopy((cast_to_fi(zeros([N*2 1],'like',real(u)))));

coder.unroll();
for ii=1:N
    temp((ii-1)*2+1) = real(u(ii));
    temp((ii-1)*2+2) = imag(u(ii));
end

y = temp;

== matlab function TxSteering_RxMVDR_4x4_HDL_IQ/DUT/Rx Beamforming/MVDR HDL/Moving Average/Window Delay/Delay Enabled Synchronous RAM Based/Zero on Initial Delay/Zeros Like ==
  settings: fimath=hdlfimath
  data: u input; y output; matchInputSize parameter; outputSize parameter
function y = zeros_like(u, matchInputSize, outputSize)

if matchInputSize
    y = zeros(size(u),'like',u);
else
    y = zeros(outputSize,'like',u);
end

== matlab function TxSteering_RxMVDR_4x4_HDL_IQ/S2MM DMA Behavioral/AXI Stream Deserializer ==
  data: data_i input; data_o output; valid_i input; valid_o output boolean; FRAME_SIZE parameter
function [data_o, valid_o] = axis_deserializer(data_i, valid_i, FRAME_SIZE)

persistent cntr bank frame_int

if isempty(cntr)
    bank = false;
    frame_int = zeros(FRAME_SIZE, 2, 'like', data_i);
    cntr = 1;
end

% default outputs
valid_o = false;
bankidx = bank;

% Latch the frame, if we're ready to send another
if valid_i
    frame_int(cntr, bankidx+1) = data_i;
    if cntr == FRAME_SIZE
        cntr = 1;
        valid_o = true;
        bank = ~bank;
    else
        cntr = cntr + 1;
    end
end

data_o = frame_int(:,bankidx+1);

== matlab function TxSteering_RxMVDR_4x4_HDL_IQ/DUT/Rx Beamforming/Output Selector/PackInput/Pack Samples/Pack Samples Fcn ==
  settings: fimath=hdlfimath;
  data: u input; y output; is_complex parameter
function y = pack_samples(u,is_complex)
%#codegen

if is_complex
    y = pack_complex(u);
else
    y = pack_real(u);
end

end

function y = pack_real(u)

    assert(isreal(u),'Expected input to be real');
    
    N = coder.const(numel(u));
    
    temp = coder.nullcopy((cast_to_fi(zeros([N 1],'like',u))));
    
    coder.unroll();
    for ii=N:-1:1
        temp(N-ii+1) = u(ii);
    end
    
    y = bitconcat(temp);

end

function y = pack_complex(u)

    assert(~isreal(u),'Expected input to be complex');
    
    N = coder.const(numel(u));
    
    temp = coder.nullcopy((cast_to_fi(zeros([N*2 1],'like',real(u)))));
    
    % Interleave real/imag
    coder.unroll();
    for ii=N:-1:1
        temp((ii-1)*2+2) = real(u(N-ii+1));
        temp((ii-1)*2+1) = imag(u(N-ii+1));
    end
    
    y = bitconcat(temp);

end

== matlab function TxSteering_RxMVDR_4x4_HDL_IQ/Software Interface Behavioral/Channel Calibration Control ==
  data: FrameData output; FrameValid output; dataIn input; TxNCOEnable output; validIn input; TxNCOInc output; MVDREnable output; RxCaptureSource output; RxCaptureTrig output; RxCalCoeffs output; NCO_default_inc parameter; state output
function [FrameData,FrameValid,TxNCOEnable,TxNCOInc,MVDREnable,...
    RxCaptureSource,RxCaptureTrig,RxCalCoeffs,state] = ...
    calibration_control(dataIn,validIn,NCO_default_inc)
% This state machine performs calibration on the Rx channels before
% entering into normal capture mode.

STATE_INIT = 0;
STATE_RUN_CAL = 1;
STATE_POSTCAL_DELAY = 2;
STATE_TRIG_CAPTURE = 3;
STATE_WAIT_VALID = 4;
STATE_DELAY = 5;

NUM_CHAN = 4;
FRAME_SIZE = length(dataIn)/NUM_CHAN;

persistent next_state next_count count_max
if isempty(next_state)
   next_state = STATE_INIT;
   next_count = 1;
   count_max = 50;
end

persistent TxNCOEnable_p MVDREnable_p RxCalCoeffs_p MVDRData_p RxCaptureSource_p
if isempty(TxNCOEnable_p)
    TxNCOEnable_p = true;
    MVDREnable_p = false;
    RxCalCoeffs_p = complex(ones(NUM_CHAN, 1));
    MVDRData_p = complex(zeros(FRAME_SIZE, 1));
    RxCaptureSource_p = fi(0, numerictype(0,2,0));
end

% update state variables
state = next_state;
count = next_count;

% output defaults
RxCaptureTrig = false;
FrameValid = false;

% state transition logic
switch state
    case STATE_INIT
        if count == count_max
            next_state = STATE_RUN_CAL;
            RxCaptureSource_p(:) = 2;
            RxCaptureTrig = true;
        else
            next_count = count + 1;
        end
    case STATE_RUN_CAL
        if validIn
            disp('Running calibration...');
            coeffs = runCal(dataIn);
            fprintf('Applying channel gains:\n');
            for ii=1:4
                fprintf('%d: scale %.2f, phase %.2f degrees\n',int32(ii),...
                    abs(coeffs(ii)),rad2deg(angle(coeffs(ii))));
            end
            RxCalCoeffs_p = coeffs;
            TxNCOEnable_p = false;
            next_state = STATE_POSTCAL_DELAY;
            next_count = 1;
            count_max = 40;
        end
    case STATE_POSTCAL_DELAY
        next_count=count+1;
        if count == count_max
            next_state = STATE_DELAY;
            MVDREnable_p = true;
            RxCaptureSource_p(:) = 0;
            next_count = 1;
            count_max = 4000;
        end
    case STATE_TRIG_CAPTURE
        next_state = STATE_WAIT_VALID;
        RxCaptureTrig = true;
    case STATE_WAIT_VALID
        if validIn
            next_state = STATE_DELAY;
            next_count = 1;
            count_max = 50;
            MVDRData_p = unpackMVDRData(dataIn);
            FrameValid = true;
        end
    case STATE_DELAY
        next_count=count+1;
        if count == count_max
            next_state = STATE_TRIG_CAPTURE;
        end
end

% outputs
TxNCOInc = NCO_default_inc;
TxNCOEnable = TxNCOEnable_p;
MVDREnable = MVDREnable_p;
RxCaptureSource = RxCaptureSource_p;
RxCalCoeffs = RxCalCoeffs_p;
FrameData = MVDRData_p;

end


function calCoeffs = runCal(dataIn)
    % Unpack uint32 to complex int16
    temp = unpack_complex(dataIn);
    % Convert to double and scale
    temp = double(temp)*2^-15;
    % Reshape into individual channels
    temp = reshape(temp,4,[]);
    % Make channels as columns
    temp = transpose(temp);
    % Get calibration coefficients
    calCoeffs = calibrate_channels(temp);
end

function dataOut = unpackMVDRData(dataIn)
    % reshape into individual channels
    temp = reshape(dataIn,4,[]);
    % grab real/imag from chan 1&2, discard chan 3&4
    temp = complex(temp(1,:), temp(2,:));
    % make channels as columns
    temp = transpose(temp);
    % Cast to fi and reinterpret fraction length
    temp = cast_to_fi(temp);
    temp = reinterpretcast(temp, numerictype(1,32,26));
    % Convert to double
    dataOut = double(temp);
end

== matlab function TxSteering_RxMVDR_4x4_HDL_IQ/DUT/Rx Beamforming/MVDR HDL/Compute Weight Vector/Serialize Input Data/readyQueue ==
  data: readyEdge input; validOut output; validIn input
function validOut = readyQueue(readyEdge, validIn)

persistent readyQueued_reg
if isempty(readyQueued_reg)
    readyQueued_reg = false;
end

readyQueued = readyQueued_reg;

if readyEdge
    if validIn
        validOut = true;
    else
        validOut = false;
        readyQueued_reg = true;
    end
elseif readyQueued
    if validIn
        validOut = true;
        readyQueued_reg = false;
    else
        validOut = false; 
    end
else
    validOut = false;
end

== matlab function TxSteering_RxMVDR_4x4_HDL_IQ/DUT/Rx Beamforming/Output Selector/PackMVDR/Pack Samples/Pack Samples Fcn ==
  settings: fimath=hdlfimath;
  data: u input; y output; is_complex parameter
function y = pack_samples(u,is_complex)
%#codegen

if is_complex
    y = pack_complex(u);
else
    y = pack_real(u);
end

end

function y = pack_real(u)

    assert(isreal(u),'Expected input to be real');
    
    N = coder.const(numel(u));
    
    temp = coder.nullcopy((cast_to_fi(zeros([N 1],'like',u))));
    
    coder.unroll();
    for ii=N:-1:1
        temp(N-ii+1) = u(ii);
    end
    
    y = bitconcat(temp);

end

function y = pack_complex(u)

    assert(~isreal(u),'Expected input to be complex');
    
    N = coder.const(numel(u));
    
    temp = coder.nullcopy((cast_to_fi(zeros([N*2 1],'like',real(u)))));
    
    % Interleave real/imag
    coder.unroll();
    for ii=N:-1:1
        temp((ii-1)*2+2) = real(u(N-ii+1));
        temp((ii-1)*2+1) = imag(u(N-ii+1));
    end
    
    y = bitconcat(temp);

end

== matlab function TxSteering_RxMVDR_4x4_HDL_IQ/Software Interface Behavioral/Display Beamforming Patterns ==
  data: computedWeights input; signalAngle input; interfererAngle input
function updatePlot(computedWeights,signalAngle,interfererAngle)

coder.extrinsic('figure','findall','close','axes','evalin','pattern',...
    'plot_beam_patterns');

persistent hAxes sensorArray steeringVector fc

if isempty(sensorArray)
    figName = coder.const('MVDR Response Pattern');
    close(findall(0,'type','figure','name',figName));
    hFig = figure('Name',figName);
    hAxes = axes(hFig);
    sensorArray = evalin('base','sensorArray');
    steeringVector = evalin('base','steeringVector');
    fc = evalin('base','fc');
end

% Compute MVDR beamformer response
mvdrWeights = double(complex(computedWeights(1:2:end),computedWeights(2:2:end)));
mvdrResponse=pattern(sensorArray,fc,-90:90,0,'Weights',mvdrWeights);

% Compute phase shift beamformer response
phaseShiftWeights=steeringVector(fc,[signalAngle; 0]);
phaseShiftResponse=pattern(sensorArray,fc,-90:90,0,'Weights',phaseShiftWeights);

% Plot beamforming patterns
plot_beam_patterns(hAxes,mvdrResponse,phaseShiftResponse,signalAngle,interfererAngle);

== matlab function TxSteering_RxMVDR_4x4_HDL_IQ/Software Interface Behavioral/Process Beam Data/QPSK Receiver ==
  data: dataIn input; FrameLength parameter size=1; SamplesPerSymbol parameter size=1; PreambleLength parameter size=1; mfCoeffs parameter; rrcCoeffs parameter; dataOut output
function dataOut = qpsk_receiver(dataIn, ...
    FrameLength, SamplesPerSymbol, PreambleLength, ...
    mfCoeffs, rrcCoeffs)

dataOut = qpsk_receive(dataIn,FrameLength,SamplesPerSymbol,PreambleLength,...
    mfCoeffs, rrcCoeffs);

== matlab function TxSteering_RxMVDR_4x4_HDL_IQ/Software Interface Behavioral/Interleave Complex 3/interleave_complex_fcn ==
  settings: fimath=hdlfimath
  data: u input; y output
function y = interleave_complex(u)
%#codegen

assert(~isreal(u),'Expected input to be complex');

N = coder.const(numel(u));

temp = coder.nullcopy((cast_to_fi(zeros([N*2 1],'like',real(u)))));

coder.unroll();
for ii=1:N
    temp((ii-1)*2+1) = real(u(ii));
    temp((ii-1)*2+2) = imag(u(ii));
end

y = temp;

== matlab function TxSteering_RxMVDR_4x4_HDL_IQ/DUT/Rx Input Preparation/Deinterleave Complex/deinterleave_complex_fcn ==
  settings: fimath=hdlfimath
  data: u input; y output
function y = deinterleave_complex(u)
%#codegen

N = coder.const(numel(u));

assert(isreal(u), 'Expected input to be real.');

temp = coder.nullcopy((cast_to_fi(complex(zeros([N/2 1],'like',u)))));

coder.unroll();
for ii=1:N/2
    temp(ii) = complex(u((ii-1)*2+1),u((ii-1)*2+2));
end

y = temp;
